simulink model "Tetraedro_model_sem_simulacao"  (R2022b)
settings: Solver=ode3  StartTime=0.0  StopTime=3000  FixedStep=.05  MaxStep=0.05  RelTol=1e-3  EnableMultiTasking=on
libraries: aerolibutil x2, sharedtransform x1, instrumentlib x1, vrlib x1
settings Model: Creator=Daniel  LastModifiedBy=labt5
settings SolverCC: AlgebraicLoopSolver=TrustRegion
settings DataIOCC: LimitDataPoints=on  SaveFormat=Array  ReturnWorkspaceOutputs=off
settings OptimizationCC: LifeSpan=inf
settings DebuggingCC: UnderspecifiedInitializationDetection=Classic  MergeDetectMultiDrivingBlocksExec=none  SolverPrmCheckMsg=warning  UnconnectedInputMsg=warning  UnconnectedOutputMsg=warning  UnconnectedLineMsg=warning  StateNameClashWarn=warning  SFUnexpectedBacktrackingDiag=warning  SFNoUnconditionalDefaultTransitionDiag=warning  SFExecutionAtInitializationDiag=none  SFMachineParentedDataDiag=warning  ArithmeticOperatorsInVariantConditions=warning
settings HardwareCC: ProdBitPerPointer=32  ProdBitPerSizeT=32  ProdBitPerPtrDiffT=32  ProdLargestAtomicFloat=None  ProdIntDivRoundTo=Undefined  ProdEndianess=Unspecified  ProdWordSize=32  ProdHWDeviceType=32-bit Generic
settings ModelReferenceCC: PropagateSignalLabelsOutOfModel=off
settings SFSimCC: SimUseLocalCustomCode=off  CustomCodeUndefinedFunction=UseInterfaceOnly
settings RTWCC: RTWUseLocalCustomCode=off
settings CodeAppCC: StateflowObjectComments=on
settings GRTTargetCC: TargetLangStandard=C89/C90 (ANSI)
settings ConfigComp: CovMetricSettings=dw  CovSaveCumulativeToWorkspaceVar=on  CovSaveSingleToWorkspaceVar=on  CovExternalEMLEnable=off
settings SimscapeCC: SimscapeNormalizeSystem=off
settings ConfigurationSet: Description=SimMechanics 2G

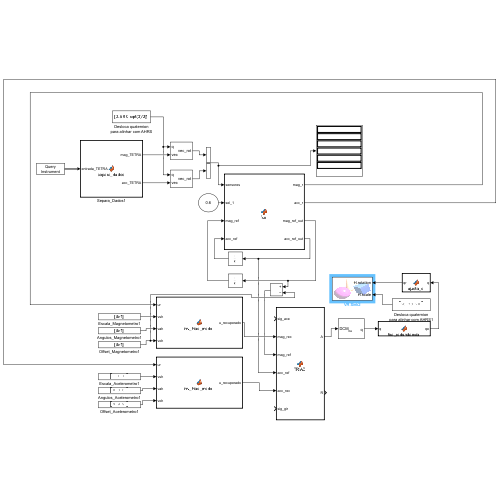
[thumbnail: Simulink's stored preview of the top-level diagram]
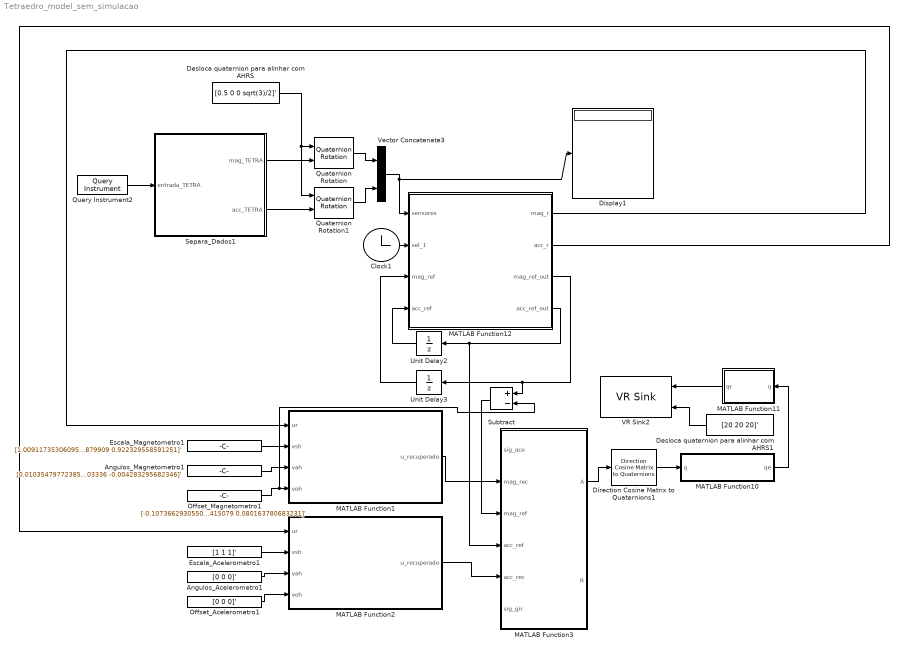
== system Tetraedro_model_sem_simulacao ==
  Angulos_Acelerometro1 : Constant  Value=[0 0 0]'
  Angulos_Magnetometro1 : Constant  Value=[0.010354797723851 -0.011935359803336 -0.004283295682346]'
  Clock1 : Clock
  Desloca quaternion para alinhar com AHRS : Constant  Value=[0.5 0 0 sqrt(3)/2]'
  Desloca quaternion para alinhar com AHRS1 : Constant  Value=[20 20 20]'
  Direction Cosine Matrix to Quaternions1 : sharedtransform/Direction Cosine Matrix  to Quaternions  aMode=aMode  action=None  tolerance=eps(2)
      settings: LibrarySourceBlock=|
      | aerolibtransform2/Direction Cosine Matrix
      | to Quaternions
  Display1 : Display
      settings: Format=binary (Stored Integer)
  Escala_Acelerometro1 : Constant  Value=[1 1 1]'
  Escala_Magnetometro1 : Constant  Value=[1.009117353060959 1.004116713879909 0.922329558591251]'
  MATLAB Function1 : MATLAB Function  TreatAsAtomicUnit=on
  MATLAB Function10 : MATLAB Function  TreatAsAtomicUnit=on
  MATLAB Function11 : MATLAB Function  TreatAsAtomicUnit=on
  MATLAB Function12 : MATLAB Function  TreatAsAtomicUnit=on
  MATLAB Function2 : MATLAB Function  TreatAsAtomicUnit=on
  MATLAB Function3 : MATLAB Function  TreatAsAtomicUnit=on
  Offset_Acelerometro1 : Constant  Value=[0 0 0]'
  Offset_Magnetometro1 : Constant  Value=[-0.107366293055073 -0.214647257415079 0.080163780683231]'
  Quaternion Rotation : aerolibutil/Quaternion Rotation
  Quaternion Rotation1 : aerolibutil/Quaternion Rotation
  Query Instrument2 : instrumentlib/Query Instrument  sampleTime=.05  isWorkspaceObject=off  timeout=5  inputBufferSize=50  protocol=Serial  serialPort=COM1  baudRate=115200  gpibVendor=Keysight Technologies  boardIndex=0  primaryAddress=1  secondaryAddress=0  visaVendor=Keysight  visaSerialPort=0  chassisIndex=0  logicalAddress=0  tcpRemoteHost='127.0.0.1'  tcpRemotePort=4500  udpRemoteHost='127.0.0.1'  udpRemotePort=9090  visaTCPBoardIndex=0  visaTCPRemoteHost='127.0.0.1'  usbBoardIndex=0  usbManufID=0  usbModelCode=0  usbSerialNumber=0  initAction=None  initCommand='DATA:SOURCE CH1'  initFunction=get  queryCommand='@'  responseFormat=ASCII  asciiFormatting='%d %d %d %d %d %d'  precision=16-bit integer  byteOrder=Little endian  valuesToRead=18  removeBytes=off  afterOutputAction=Repeat query for new data  enableFrames=on  frameSize=6
  Separa_Dados1 : MATLAB Function  TreatAsAtomicUnit=on
  Subtract : Sum  Inputs=+-
  Unit Delay2 : UnitDelay  InitialCondition=[0 0 0]'  SampleTime=-1  HasFrameUpgradeWarning=on
  Unit Delay3 : UnitDelay  InitialCondition=[0 0 0]'  SampleTime=-1  HasFrameUpgradeWarning=on
  VR Sink2 : vrlib/VR Sink  InstantiateOnLoad=on  SampleTime=-1  ViewEnable=on  RemoteChange=off  RemoteView=off  FieldsWritten=H.rotation.4.1.1.double#H.scale.3.1.1.double  WorldFileName=C:\Users\labt5\OneDrive\Desktop\Cesar\IC_2024_Cesar\Matlab\simulink\Arquivos WRL\teste_combinado.wrl  AutoView=off  VideoDimensions=[]  AllowVariableSize=off
  Vector Concatenate3 : Concatenate
  wires:
  Offset_Magnetometro1/1 -> Subtract/2, MATLAB Function1/4(voh)
  Escala_Acelerometro1/1 -> MATLAB Function2/2(vsh)
  Angulos_Acelerometro1/1 -> MATLAB Function2/3(vah)
  Offset_Acelerometro1/1 -> MATLAB Function2/4(voh)
  Escala_Magnetometro1/1 -> MATLAB Function1/2(vsh)
  Angulos_Magnetometro1/1 -> MATLAB Function1/3(vah)
  MATLAB Function2/1(u_recuperado) -> MATLAB Function3/5(acc_rec)
  MATLAB Function1/1(u_recuperado) -> MATLAB Function3/2(mag_rec)
  MATLAB Function3/1(A) -> Direction Cosine Matrix to Quaternions1/1
  Direction Cosine Matrix to Quaternions1/1 -> MATLAB Function10/1(q)
  Unit Delay2/1 -> MATLAB Function12/4(acc_ref)
  Unit Delay3/1 -> MATLAB Function12/3(mag_ref)
  MATLAB Function12/3(mag_ref_out) -> Subtract/1, Unit Delay3/1
  MATLAB Function12/4(acc_ref_out) -> Unit Delay2/1, MATLAB Function3/4(acc_ref)
  Clock1/1 -> MATLAB Function12/2(sel_1)
  MATLAB Function12/1(mag_r) -> MATLAB Function1/1(ur)
  MATLAB Function12/2(acc_r) -> MATLAB Function2/1(ur)
  MATLAB Function10/1(qe) -> MATLAB Function11/1(q)
  Query Instrument2/1 -> Separa_Dados1/1(entrada_TETRA)
  Separa_Dados1/1(mag_TETRA) -> Quaternion Rotation/2
  Separa_Dados1/2(acc_TETRA) -> Quaternion Rotation1/2
  Desloca quaternion para alinhar com AHRS/1 -> Quaternion Rotation1/1, Quaternion Rotation/1
  Quaternion Rotation/1 -> Vector Concatenate3/1
  Quaternion Rotation1/1 -> Vector Concatenate3/2
  Vector Concatenate3/1 -> Display1/1, MATLAB Function12/1(sensores)
  Subtract/1 -> MATLAB Function3/3(mag_ref)
  MATLAB Function11/1(qr) -> VR Sink2/1
  Desloca quaternion para alinhar com AHRS1/1 -> VR Sink2/2

== matlab function Tetraedro_model_sem_simulacao/MATLAB Function1 ==
  data: ur input; u_recuperado output; vsh input; vah input; voh input
function u_recuperado = inv_triad_model(ur,vsh,vah,voh)
%#eml

rho = vah(1);
phi = vah(2);
lambda = vah(3);

T_inv = [1 0 0; -tan(rho) 1/cos(rho) 0;...
    tan(rho)*tan(lambda)-tan(phi) -tan(lambda)/cos(rho) 1/(cos(lambda)*cos(phi))];
S_inv = inv(diag(vsh));

u_recuperado = T_inv*S_inv*(ur - voh);

== matlab function Tetraedro_model_sem_simulacao/MATLAB Function10 ==
  data: q input; qe output
function qe = tira_redundancia(q)
qe = zeros(4,1);
%#eml

if q(1)<0
    qe = -q;
else
    qe = q;
end

== matlab function Tetraedro_model_sem_simulacao/MATLAB Function11 ==
  data: q input; qr output
function qr = ajusta_q(q)
%#eml

q = q/(norm(q));
v = [q(2) q(3) q(4)] / norm([q(2) q(3) q(4)]);
ang = acos(q(1))*2;

qr = [v ang];

== matlab function Tetraedro_model_sem_simulacao/MATLAB Function12 ==
  data: sensores input; sel_1 input; mag_r output; acc_r output; mag_ref input; acc_ref input; mag_ref_out output; acc_ref_out output
function [mag_r, acc_r, mag_ref_out, acc_ref_out] = fcn(sensores, sel_1, mag_ref, acc_ref)
%#codegen

mag_ref_out = zeros(3,1);
acc_ref_out = zeros(3,1);

mag_x = sensores(1);
mag_y = sensores(2);
mag_z = sensores(3);

acc_x = sensores(4);
acc_y = sensores(5);
acc_z = sensores(6);

mag_ref_out = mag_ref;
acc_ref_out = acc_ref;

if sel_1 == 0
mag_ref_out = [mag_x mag_y mag_z]';
acc_ref_out = [acc_x acc_y acc_z]';
end

mag_r = [mag_x mag_y mag_z]';
acc_r = [acc_x acc_y acc_z]';

== matlab function Tetraedro_model_sem_simulacao/MATLAB Function2 ==
  data: ur input; u_recuperado output; vsh input; vah input; voh input
function u_recuperado = inv_triad_model(ur,vsh,vah,voh)
%#eml

rho = vah(1);
phi = vah(2);
lambda = vah(3);

T_inv = [1 0 0; -tan(rho) 1/cos(rho) 0;...
    tan(rho)*tan(lambda)-tan(phi) -tan(lambda)/cos(rho) 1/(cos(lambda)*cos(phi))];
S_inv = inv(diag(vsh));

u_recuperado = T_inv*S_inv*(ur - voh);

== matlab function Tetraedro_model_sem_simulacao/MATLAB Function3 ==
  data: sig_ace input; A output; mag_rec input; mag_ref input; acc_ref input; acc_rec input; sig_gir input; R output
function [A,R] = TRIAD(sig_ace,mag_rec,mag_ref,acc_ref,acc_rec,sig_gir)

% ========== Função de Determinação de Atitude ===========
% ========== Algoritmo TRIAD ===========
% Os parâmetros de Entrada são:
% V1 : vetor de referência V1
V1 = acc_ref;
% V2 : vetor de referência V2
V2 = mag_ref;
% W1 : vetor de observação W1
W1 = acc_rec;
% W2 : vetor de observação W2
W2 = mag_rec;
% SigTo1 : desvio padrão das observação do Acelerômetro
SigTot1 = sig_ace;
% SigTo2 : desvio padrão das observação do Magnetômetro
SigTot2 = sig_gir;

% ========================================================
% Os parâmetros de Retorno são:
% A : matriz de atitude
% P : Covariância da atitude
% ========================================================
% --- Obtendo a Tríade de Referência
r1 = V1/norm(V1);
r2 = cross(V1,V2); % função do produto vetorial
r2 = r2 / norm(r2);
r3 = cross(r1,r2);
% --- Montando a Matriz de Referência
Mref = [r1 r2 r3];

% --- Obtendo a tríade de observação
s1 = W1/norm(W1);
s2 = cross(W1,W2);
s2 = s2 / norm(s2);
s3 = cross(s1,s2);
% --- Montando a Matriz de Observação
Mobs = [s1 s2 s3];
% --- Atitude pelo TRIAD
A = Mobs * Mref';
%--------------------------------------------------------------------------
% Obtendo a covariância da atitude (P = P + AP AT)
R = SigTot1^2 * eye(3) + ...
    (1/norm(cross(W1,W2)))^2 * (SigTot1^2* (W1'*W2) * (W1*W2' + W2*W1')...
    + (SigTot2^2 - SigTot1^2)*W1*W1');

%--------------------------------------------------------------------------

== matlab function Tetraedro_model_sem_simulacao/Separa_Dados1 ==
  data: mag_TETRA output; entrada_TETRA input; acc_TETRA output
function [mag_TETRA, acc_TETRA]  = separa_dados(entrada_TETRA)
%#codegen

mag_TETRA = zeros(3,1);
acc_TETRA = zeros(3,1);

mag_x = entrada_TETRA(1);
mag_y = entrada_TETRA(2);
mag_z = entrada_TETRA(3);

acc_x = entrada_TETRA(4);
acc_y = entrada_TETRA(5);
acc_z = entrada_TETRA(6);


mag_TETRA = [mag_x mag_y mag_z]';
acc_TETRA = [acc_x acc_y acc_z]';
